simulink model "sim1"  (R2023a)
settings: Solver=VariableStepAuto  StartTime=0  StopTime=7  FixedStep=0.01  RelTol=1e-8
undefined symbols (not defined in the file): a0, a1, dy0, sw, y0
libraries: simulink x1
settings Model: Creator=vasil  LastModifiedBy=vasil

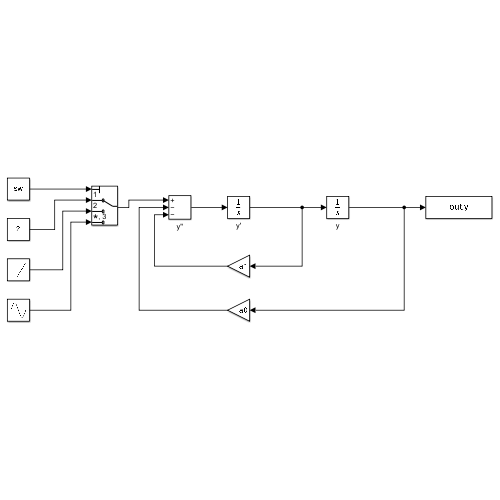
[thumbnail: Simulink's stored preview of the top-level diagram]
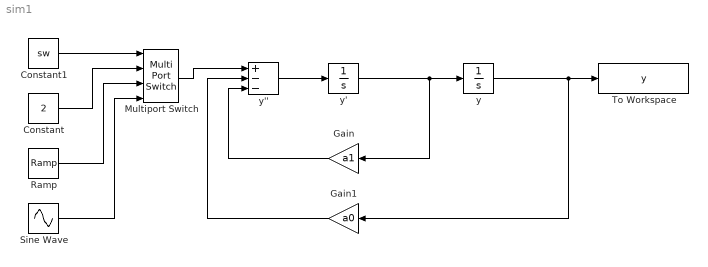
== system sim1 ==
  Constant : Constant  Value=2
  Constant1 : Constant  Value=sw
  Gain : Gain  Gain=a1
  Gain1 : Gain  Gain=a0
  Multiport Switch : MultiPortSwitch  SaturateOnIntegerOverflow=off  InputSameDT=off
  Ramp : simulink/Sources/Ramp  slope=0.7  start=0  InitialOutput=0
  Sine Wave : Sin  Frequency=7  SampleTime=0
  To Workspace : ToWorkspace  VariableName=y  SaveFormat=Timeseries  SampleTime=-1
  y : Integrator  InitialCondition=y0
  y' : Integrator  InitialCondition=dy0
  y'' : Sum  Inputs=+--
  wires:
  y/1 -> Gain1/1, To Workspace/1
  y''/1 -> y'/1
  Gain1/1 -> y''/2
  y'/1 -> Gain/1, y/1
  Gain/1 -> y''/3
  Multiport Switch/1 -> y''/1
  Constant1/1 -> Multiport Switch/1
  Constant/1 -> Multiport Switch/2
  Ramp/1 -> Multiport Switch/3
  Sine Wave/1 -> Multiport Switch/4
